simulink model "Main_Simulation_2020a"  (R2020a)
settings: Solver=ode45  StartTime=0.0  StopTime=200  MaxStep=0.01  RelTol=1e-7
values from neighbouring files (symbols this model uses):
  beta = 10    [parameters.m]
  I_g = diag([0.13, 0.16, 0.2])    [parameters.m]
  k1 = 1    [parameters.m]
  k2 = 2    [parameters.m]
  K_p = 10    [parameters.m]
  kp = 16    [parameters.m]
  kv = 6    [parameters.m]
  L = [-(1/2)^(-1/2) -(1/2)^(-1/2) (1/2)^(-1/2)  (1/2)^(-1/2) 0 0 0 0 ... (first row only)    [parameters.m]
  m = 10    [parameters.m]
  M_11 = MRB_11 + MA_11    [parameters.m]
  M_22 = MRB_22 + MA_22    [parameters.m]
  M_q = 10    [parameters.m]
  N_r = 10    [parameters.m]
  r_g = [0 0 0]'    [parameters.m]
  X_u = 10    [parameters.m]
  Y_v = 10    [parameters.m]
  Z_w = 10    [parameters.m]
settings Model: Creator=edward  LastModifiedBy=edward

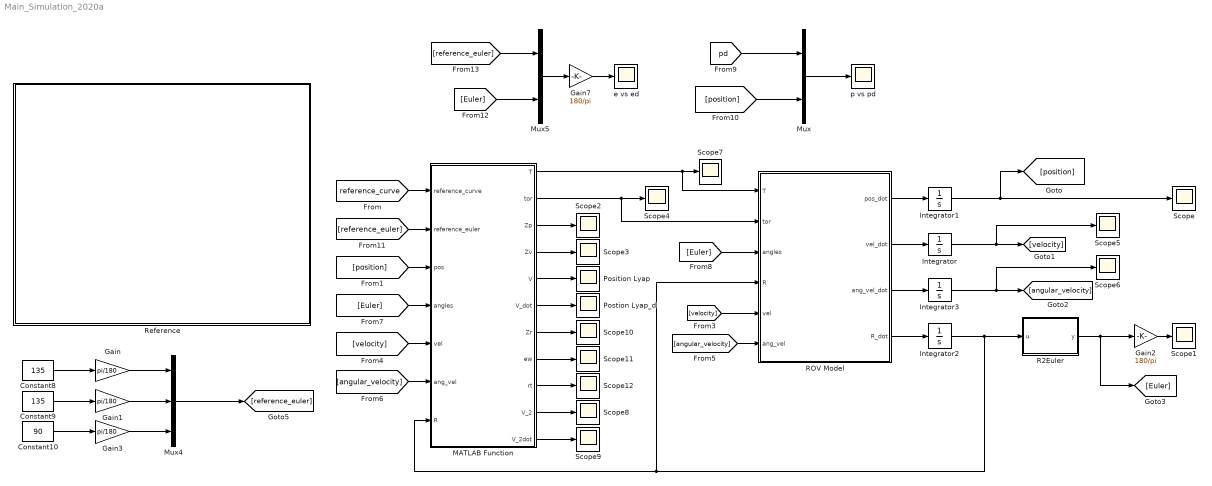
== system Main_Simulation_2020a ==
  Constant10 : Constant  Value=90
  Constant8 : Constant  Value=135
  Constant9 : Constant  Value=135
  Gain : Gain  Gain=pi/180
  Gain1 : Gain  Gain=pi/180
  Gain2 : Gain  Gain=180/pi
  Gain3 : Gain  Gain=pi/180
  Gain7 : Gain  Gain=180/pi
  Integrator : Integrator  InitialCondition=zeros(3,1)
  Integrator1 : Integrator  InitialCondition=[100; 50; -25]
  Integrator2 : Integrator  InitialCondition=eye(3)
  Integrator3 : Integrator  InitialCondition=zeros(3,1)
  MATLAB Function : MATLAB Function  TreatAsAtomicUnit=on
  Mux : Mux  Inputs=2
  Mux4 : Mux  Inputs=3
  Mux5 : Mux  Inputs=2
  Position Lyap : Scope
  Postion Lyap_d : Scope
  R2Euler : MATLAB Function  TreatAsAtomicUnit=on
  ROV Model : MATLAB Function  TreatAsAtomicUnit=on
  Reference : Subsystem
  Scope{,1..12} (13 alike) : Scope
  e vs ed : Scope
  p vs pd : Scope
  wires:
  ROV Model/2(vel_dot) -> Integrator/1
  ROV Model/1(pos_dot) -> Integrator1/1
  Integrator1/1 -> [position], Scope/1
  ROV Model/4(R_dot) -> Integrator2/1
  Integrator2/1 -> R2Euler/1(u), ROV Model/4(R), MATLAB Function/7(R)
  R2Euler/1(y) -> Gain2/1, [Euler]
  Gain2/1 -> Scope1/1
  MATLAB Function/1(T) -> Scope7/1, ROV Model/1(T)
  Integrator/1 -> Scope5/1, [velocity]
  MATLAB Function/3(Zp) -> Scope2/1
  [reference_curve] -> MATLAB Function/1(reference_curve)
  ROV Model/3(ang_vel_dot) -> Integrator3/1
  [position] -> MATLAB Function/3(pos)
  [velocity] -> ROV Model/5(vel)
  [velocity] -> MATLAB Function/5(vel)
  [angular_velocity] -> ROV Model/6(ang_vel)
  [angular_velocity] -> MATLAB Function/6(ang_vel)
  [Euler] -> ROV Model/3(angles)
  [Euler] -> MATLAB Function/4(angles)
  [pd] -> Mux/1
  [position] -> Mux/2
  Mux/1 -> p vs pd/1
  MATLAB Function/5(V) -> Position Lyap/1
  MATLAB Function/4(Zv) -> Scope3/1
  Integrator3/1 -> Scope6/1, [angular_velocity]
  MATLAB Function/6(V_dot) -> Postion Lyap_d/1
  MATLAB Function/2(tor) -> Scope4/1, ROV Model/2(tor)
  Constant8/1 -> Gain/1
  Constant9/1 -> Gain1/1
  Constant10/1 -> Gain3/1
  Gain/1 -> Mux4/1
  Gain1/1 -> Mux4/2
  Gain3/1 -> Mux4/3
  Mux4/1 -> [reference_euler]
  [reference_euler] -> MATLAB Function/2(reference_euler)
  Mux5/1 -> Gain7/1
  [Euler] -> Mux5/2
  [reference_euler] -> Mux5/1
  MATLAB Function/10(V_2) -> Scope8/1
  MATLAB Function/11(V_2dot) -> Scope9/1
  MATLAB Function/7(Zr) -> Scope10/1
  Gain7/1 -> e vs ed/1
  MATLAB Function/8(ew) -> Scope11/1
  MATLAB Function/9(rt) -> Scope12/1

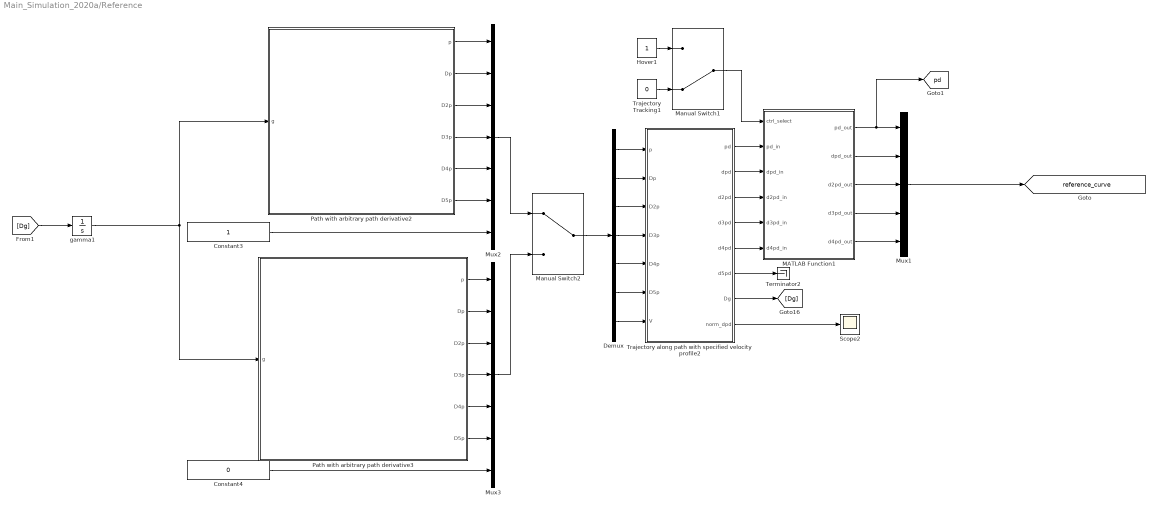
== system Main_Simulation_2020a/Reference ==
  Constant3 : Constant
  Constant4 : Constant  Value=0
  Demux : Demux  Outputs=7
  Hover1 : Constant
  MATLAB Function1 : MATLAB Function  TreatAsAtomicUnit=on
  Manual Switch1 : ManualSwitch  CurrentSetting=0
  Manual Switch2 : ManualSwitch
  Mux1 : Mux  Inputs=5
  Mux2 : Mux  Inputs=7
  Mux3 : Mux  Inputs=7
  Path with arbitrary path derivative2 : MATLAB Function  TreatAsAtomicUnit=on  mask{ra=10, rb=10, a=3, b=3, delta=pi/2, h=0, f=0}
      mask prompts: ra "A"; rb "B"; h "Mean height"; f "Height frequency"
      mask help:
      | x=A*sin(a*g+delta)
      | y=B*sin(b*g)
  Path with arbitrary path derivative3 : MATLAB Function  TreatAsAtomicUnit=on  mask{va=0, h=0}
      mask prompts: va "Radius"; h "Height"
      mask help:
      | x = va*(1 + cos(g))
      | y = va*sin(g)
      | z = 2*va*sin(g/2)
  Scope2 : Scope
  Terminator2 : Terminator
  Trajectory Tracking1 : Constant  Value=0
  Trajectory along path with specified velocity profile2 : MATLAB Function  TreatAsAtomicUnit=on
  gamma1 : Integrator
  tag scope: pd=global, reference_curve=global
  wires:
  Trajectory along path with specified velocity profile2/5(d4pd) -> MATLAB Function1/6(d4pd_in)
  Demux/5 -> Trajectory along path with specified velocity profile2/5(D4p)
  Path with arbitrary path derivative2/5(D4p) -> Mux2/5
  Constant3/1 -> Mux2/7
  MATLAB Function1/2(dpd_out) -> Mux1/2
  MATLAB Function1/3(d2pd_out) -> Mux1/3
  MATLAB Function1/1(pd_out) -> [pd], Mux1/1
  Trajectory along path with specified velocity profile2/2(dpd) -> MATLAB Function1/3(dpd_in)
  Path with arbitrary path derivative2/3(D2p) -> Mux2/3
  Demux/6 -> Trajectory along path with specified velocity profile2/6(D5p)
  MATLAB Function1/4(d3pd_out) -> Mux1/4
  Demux/1 -> Trajectory along path with specified velocity profile2/1(p)
  Trajectory along path with specified velocity profile2/3(d2pd) -> MATLAB Function1/4(d2pd_in)
  Path with arbitrary path derivative3/6(D5p) -> Mux3/6
  Trajectory along path with specified velocity profile2/4(d3pd) -> MATLAB Function1/5(d3pd_in)
  Trajectory along path with specified velocity profile2/1(pd) -> MATLAB Function1/2(pd_in)
  gamma1/1 -> Path with arbitrary path derivative2/1(g), Path with arbitrary path derivative3/1(g)
  MATLAB Function1/5(d4pd_out) -> Mux1/5
  Path with arbitrary path derivative2/6(D5p) -> Mux2/6
  Constant4/1 -> Mux3/7
  Path with arbitrary path derivative3/4(D3p) -> Mux3/4
  Trajectory Tracking1/1 -> Manual Switch1/2
  Manual Switch2/1 -> Demux/1
  Demux/2 -> Trajectory along path with specified velocity profile2/2(Dp)
  Demux/4 -> Trajectory along path with specified velocity profile2/4(D3p)
  Mux3/1 -> Manual Switch2/2
  Mux2/1 -> Manual Switch2/1
  Trajectory along path with specified velocity profile2/8(norm_dpd) -> Scope2/1
  Path with arbitrary path derivative3/3(D2p) -> Mux3/3
  Trajectory along path with specified velocity profile2/7(Dg) -> [Dg]
  Hover1/1 -> Manual Switch1/1
  Demux/3 -> Trajectory along path with specified velocity profile2/3(D2p)
  Path with arbitrary path derivative2/2(Dp) -> Mux2/2
  Trajectory along path with specified velocity profile2/6(d5pd) -> Terminator2/1
  Path with arbitrary path derivative3/2(Dp) -> Mux3/2
  Path with arbitrary path derivative3/1(p) -> Mux3/1
  Path with arbitrary path derivative2/1(p) -> Mux2/1
  Manual Switch1/1 -> MATLAB Function1/1(ctrl_select)
  [Dg] -> gamma1/1
  Demux/7 -> Trajectory along path with specified velocity profile2/7(V)
  Path with arbitrary path derivative2/4(D3p) -> Mux2/4
  Path with arbitrary path derivative3/5(D4p) -> Mux3/5
  Mux1/1 -> [reference_curve]

== matlab function Main_Simulation_2020a/Reference/MATLAB Function1 ==
  data: ctrl_select input; pd_out output; pd_in input; dpd_in input; d2pd_in input; d3pd_in input; d4pd_in input; dpd_out output; d2pd_out output; d3pd_out output; d4pd_out output
function [pd_out, dpd_out, d2pd_out, d3pd_out, d4pd_out] = hover_ref(ctrl_select,pd_in, dpd_in, d2pd_in, d3pd_in, d4pd_in)

pd_out      = (1 - ctrl_select)*pd_in;
dpd_out     = (1 - ctrl_select)*dpd_in;
d2pd_out    = (1 - ctrl_select)*d2pd_in;
d3pd_out    = (1 - ctrl_select)*d3pd_in;
d4pd_out    = (1 - ctrl_select)*d4pd_in;
    
if ctrl_select == 1
    pd_out(3) = -1.7;
end

== matlab function Main_Simulation_2020a/Reference/Path with arbitrary path derivative2 ==
  data: g input; ra parameter; rb parameter; a parameter; b parameter; delta parameter; p output; Dp output; D2p output; D3p output; D4p output; D5p output; h parameter size=1; f parameter
function [p,Dp,D2p,D3p,D4p,D5p] = path(g,ra,rb,a,b,delta,h,f)
%#codegen

% syms a b g delta ra rb
% p = [ra*sin(a*g+delta)/(sin(b*g)^2+1);
%      rb*sin(b*g)/(sin(b*g)^2+1)]
% diff(p,g)
% diff(p,g,2)
% diff(p,g,3)

p = [ra*sin(a*g+delta);
     rb*sin(b*g);
     h + 0.5*sin(f*g)];
 
Dp = [a*ra*cos(delta + a*g);
      b*rb*cos(b*g);
      0.5*f*cos(f*g)];
      
D2p = [-a^2*ra*sin(delta + a*g);
       -b^2*rb*sin(b*g);
       -0.5*f^2*sin(f*g)];
 
D3p = [-a^3*ra*cos(delta + a*g);
       -b^3*rb*cos(b*g);
       -0.5*f^3*cos(f*g)];
     
D4p = [a^4*ra*sin(delta + a*g);
       b^4*rb*sin(b*g);
       0.5*f^4*sin(f*g)];
 
D5p = [a^5*ra*cos(delta + a*g);
       b^5*rb*cos(b*g);
       0.5*f^5*cos(f*g)];

== matlab function Main_Simulation_2020a/Reference/Path with arbitrary path derivative3 ==
  data: g input; p output; Dp output; D2p output; D3p output; D4p output; D5p output; va parameter size=1; h parameter
function [p,Dp,D2p,D3p,D4p,D5p] = path(g,va, h)
%#codegen

% syms g va
% p = [va*sin(g);
%      2*va*sin(g/2);
%      va*(1 + cos(g))];
% diff(p,g)
% diff(p,g,2)
% diff(p,g,3)

p = [va*sin(g);
     2*va*sin(g/2);
     va*(1 + cos(g)) - h];

Dp = [va*cos(g);
       va*cos(g/2);
       -va*sin(g)];
         
D2p = [-va*sin(g);
       -(va/2)*sin(g/2);
       -va*cos(g)];

D3p = [-va*cos(g);
       -(va/4)*cos(g/2);
       va*sin(g)];
        
D4p = [va*sin(g);
       (va/8)*sin(g/2);
       va*cos(g)];
    
D5p = [va*cos(g);
        (va/16)*cos(g/2);
        -va*sin(g)];

== matlab function Main_Simulation_2020a/Reference/Trajectory along path with specified velocity profile2 ==
  data: pd output size=3; dpd output size=3; d2pd output size=3; d3pd output; d4pd output; d5pd output; Dg output; p input size=3; Dp input size=3; D2p input size=3; D3p input size=3; D4p input size=3; D5p input size=3; V input; norm_dpd output
function [pd,dpd,d2pd,d3pd,d4pd,d5pd,Dg,norm_dpd] = trajectory(p,Dp,D2p,D3p,D4p,D5p,V)
%#codegen

norm_Dp = norm(Dp);

% Parameter velocity is V times the inverse of the 
% norm of path derivative with respect to the parameter
Dg = V/norm_Dp;

% Checked
D2g = -V*(Dp'*D2p)/norm_Dp^3*Dg;

% Checked
D3g = -V/norm_Dp^3*((Dp'*D2p)*D2g + Dg^2*(norm(D2p)^2 + Dp'*D3p - 3*(Dp'*D2p)^2/norm_Dp^2));

% Checked
Aux = 2*(     (Dp'*D2p)*Dg*norm(D2p)^2/norm_Dp^2 ...
            + (Dp'*D2p)*(Dp'*D3p)*Dg/norm_Dp^2 ...
            - (Dp'*D2p)^3*Dg/norm_Dp^4);

% As seen before, Aux variable is divided into 3 different components
% In the next step, we compute the derivative of each component 

% Checked
J1 = ((norm(D2p)^2*Dg^2 + (Dp'*D3p)*Dg^2 + (Dp'*D2p)*D2g))*norm(D2p)^2/norm_Dp^2 ...
        + (Dp'*D2p)*Dg*(2*(D3p'*D2p)*Dg*norm_Dp^2 - 2*norm(D2p)^2*(D2p'*Dp)*Dg)/norm_Dp^4;

% Checked
J2_aux = norm(D2p)^2*(Dp'*D3p)*Dg^2 + (Dp'*D3p)^2*Dg^2 + (Dp'*D2p)*(D2p'*D3p)*Dg^2 + (Dp'*D2p)*(Dp'*D4p)*Dg^2 + (Dp'*D2p)*(Dp'*D3p)*D2g;

% Checked
J2 = -2*(D2p'*Dp)*Dg/norm_Dp^4*(Dp'*D2p)*(Dp'*D3p)*Dg + 1/norm_Dp^2*(J2_aux);

% Checked
J3 = -1/norm_Dp^4*(3*(Dp'*D2p)^2*(norm(D2p)^2 + (Dp'*D3p))*Dg^2 + (Dp'*D2p)^3*D2g - 4*(Dp'*D2p)^4*Dg^2/norm_Dp^2);

% Checked
Aux_der = 2*(J1 + J2 + J3);

% Checked
D4g_aux1 = (Dp'*D2p)*D2g + Dg^2*(norm(D2p)^2 + Dp'*D3p - 3*(Dp'*D2p)^2/norm_Dp^2);

% Checked
D4g_aux2 = (norm(D2p)^2 + Dp'*D3p)*D2g*Dg ... % T1
            + (Dp'*D2p)*D3g ... % T2
            +2*Dg*D2g*(norm(D2p)^2 + Dp'*D3p - 3*(Dp'*D2p)^2/norm_Dp^2) ... % T3
            +Dg^2*(2*(D3p'*D2p)*Dg + (D2p'*D3p)*Dg + (Dp'*D4p)*Dg - 3*Aux);

% Checked
D4g = 3*V*(Dp'*D2p)*Dg/norm_Dp^5*D4g_aux1 - V/norm_Dp^3*D4g_aux2;

% Checked
D4g_aux1_der = (norm(D2p)^2 + Dp'*D3p)*D2g*Dg + (Dp'*D2p)*D3g ...
                + 2*Dg*D2g*(norm(D2p)^2 + Dp'*D3p - 3*(Dp'*D2p)^2/norm_Dp^2) ...
                + Dg^2*(2*(D3p'*D2p)*Dg + (D2p'*D3p)*Dg + (Dp'*D4p)*Dg - 3*Aux);

% Checked
T1_der = (2*(D3p'*D2p)*Dg + (D2p'*D3p)*Dg + (Dp'*D4p)*Dg)*D2g*Dg + (norm(D2p)^2 + Dp'*D3p)*(D3g*Dg + D2g^2);

% Checked
T2_der = norm(D2p)^2*D3g*Dg + (Dp'*D3p)*D3g*Dg + (Dp'*D2p)*D4g;

% Checked
T3_der = 2*(D2g^2 + Dg*D3g)*(norm(D2p)^2 + Dp'*D3p - 3*(Dp'*D2p)^2/norm_Dp^2)...
        + 2*Dg*D2g*(2*(D3p'*D2p)*Dg + (D2p'*D3p)*Dg + (Dp'*D4p)*Dg - 3*Aux);

% Checked
T4_der = 2*Dg*D2g*(2*(D3p'*D2p)*Dg + (D2p'*D3p)*Dg + (Dp'*D4p)*Dg - 3*Aux) ...
            + Dg^2*(3*(D4p'*D2p)*Dg^2 + 3*norm(D3p)^2*Dg^2 + 3*D3p'*D2p*D2g + (D2p'*D4p)*Dg^2 + Dp'*D5p*Dg^2 + Dp'*D4p*D2g - 3*Aux_der);

% Checked
D4g_aux2_der = T1_der + T2_der + T3_der + T4_der;
  
D5g =   3*V*((norm(D2p)^2*Dg^2 + Dp'*D3p*Dg^2 + Dp'*D2p*D2g)/norm_Dp^5 ...
        - 5*((Dp'*D2p)^2*Dg^2)/norm_Dp^7)*D4g_aux1 ...
        + 3*V*(Dp'*D2p)*Dg/norm_Dp^5*D4g_aux1_der + 3*V*(Dp'*D2p)*Dg/norm_Dp^5*D4g_aux2 ...
        -V/norm_Dp^3*D4g_aux2_der;
    
pd      = p;
dpd     = Dp*Dg;
d2pd    = D2p*Dg^2 + Dp*D2g;
d3pd    = D3p*Dg^3 + 3*D2p*D2g*Dg + Dp*D3g;
d4pd    = D4p*Dg^4 + 6*D3p*Dg^2*D2g + D2p*(4*D3g*Dg + 3*D2g^2) + Dp*D4g;
d5pd    = D5p*Dg^5 + 10*D4p*Dg^3*D2g + 15*D3p*D2g^2*Dg + 10*D3p*Dg^2*D3g + 5*D2p*D4g*Dg + 10*D2p*D3g*D2g + Dp*D5g;

norm_dpd = norm(dpd);

== matlab function Main_Simulation_2020a/ROV Model ==
  data: T input size=3; tor input size=3; pos_dot output size=3; angles input size=3; R input; vel_dot output size=3; ang_vel_dot output size=3; vel input size=3; R_dot output size=[3 3]; ang_vel input size=3; L parameter size=[6 8]; M_11 parameter size=[3 3]; M_22 parameter size=[3 3]; I_g parameter size=[3 3]; r_g parameter size=3; X_u parameter size=1; Y_v parameter size=1; Z_w parameter size=1; K_p parameter size=1; M_q parameter size=1; N_r parameter size=1; m parameter size=1
function [pos_dot,vel_dot,ang_vel_dot,R_dot] = fcn(T,tor,angles,R,vel,ang_vel,L,M_11,M_22,I_g,r_g,X_u,Y_v,Z_w, K_p, M_q, N_r, m)

roll = angles(1);
pitch = angles(2);
yaw = angles(3);

v_surge = vel(1);
v_sway = vel(2);
v_heave = vel(3);

w_roll = ang_vel(1);
w_pitch = ang_vel(2);
w_yaw = ang_vel(3);


CRB_11 = zeros(3,3);
CRB_12 = -m*Skew(vel)-m*Skew(Skew(ang_vel)*r_g);
CRB_21 = -m*Skew(vel)-m*Skew(Skew(ang_vel)*r_g);
CRB_22 = m*Skew(Skew(vel)*r_g)-Skew(I_g*ang_vel);
   
aux_a = diag([X_u, Y_v, Z_w])*vel;
aux_b = diag([K_p, M_q, N_r])*ang_vel;

CA_11 = zeros(3,3);
CA_12 = Skew(aux_a);
CA_21 = Skew(aux_a);
CA_22 = Skew(aux_b);

C_11 = CRB_11 + CA_11;
C_12 = CRB_12 + CA_12;
C_21 = CRB_21 + CA_21;
C_22 = CRB_22 + CA_22;

Xu = 10;
Yv = 10;
Zw = 10;
Kp = 10;
Mq = 10;
Nr = 10;
Xuu = 10;
Yvv = 10;
Zww = 10;
Kpp = 10;
Mqq = 10;
Nrr = 10; 

Dl_11 = diag([Xu, Yv, Zw]);
Dl_22 = diag([Kp, Mq, Nr]);

Dq_11 = diag([Xuu*abs(v_surge), Yvv*abs(v_sway), Zww*abs(v_heave)]);
Dq_22 = diag([Kpp*abs(w_roll), Mqq*abs(w_pitch), Nrr*abs(w_yaw)]);

D_11 = Dl_11 + Dq_11;
D_22 = Dl_22 + Dq_22;


W = 9.81*m;
B = 1000*9.81*0.0480;
g_v = (W-B)*[sin(pitch);
     -cos(pitch)*sin(roll);
     -cos(pitch)*cos(roll)];

pos_dot = R*vel;

R_dot = R*Skew(ang_vel);

vel_dot = M_11\(T - [C_11 C_12]*[vel; ang_vel] - D_11*vel - g_v);

ang_vel_dot = M_22\(tor - [C_21 C_22]*[vel; ang_vel] - D_22*ang_vel);

== matlab function Main_Simulation_2020a/R2Euler ==
  data: u input; y output
function y = fcn(u)
y = rotm2eul(u, 'XYZ')';

== matlab function Main_Simulation_2020a/MATLAB Function ==
  data: reference_curve input size=15; reference_euler input size=3; pos input size=3; angles input size=3; vel input size=3; ang_vel input size=3; R input size=[3 3]; T output size=3; tor output size=3; Zp output size=3; Zv output; V output size=1; M_11 parameter size=[3 3]; m parameter size=1; M_q parameter size=1; N_r parameter size=1; r_g parameter size=3; X_u parameter size=1; Y_v parameter size=1; Z_w parameter size=1; I_g parameter size=[3 3]; K_p parameter size=1; k1 parameter size=1; k2 parameter size=1; kp parameter size=1; kv parameter size=1; beta parameter size=1; V_dot output size=1; Zr output size=[3 3]; ew output; rt output; V_2 output size=1; M_22 parameter size=[3 3]; V_2dot output size=1
function [T,tor,Zp,Zv,V,V_dot,Zr,ew,rt,V_2,V_2dot] = fcn(reference_curve,reference_euler,pos,angles,vel,ang_vel,R,M_11,m, M_q, N_r, r_g, X_u, Y_v, Z_w, I_g, K_p, k1, k2, kp, kv, beta, M_22)

pd      = reference_curve(1:3);
dpd     = reference_curve(4:6);
d2pd    = reference_curve(7:9);

roll = angles(1);
pitch = angles(2);

Zp = pos - pd;
Zv = R*vel - dpd;

v_surge = vel(1);
v_sway = vel(2);
v_heave = vel(3);

w_roll = ang_vel(1);
w_pitch = ang_vel(2);
w_yaw = ang_vel(3);

CRB_11 = zeros(3,3);
CRB_12 = -m*Skew(vel)-m*Skew(Skew(ang_vel)*r_g);
CRB_21 = -m*Skew(vel)-m*Skew(Skew(ang_vel)*r_g);
CRB_22 = m*Skew(Skew(vel)*r_g)-Skew(I_g*ang_vel);
   
aux_a = diag([X_u, Y_v, Z_w])*vel;
aux_b = diag([K_p, M_q, N_r])*ang_vel;

CA_11 = zeros(3,3);
CA_12 = Skew(aux_a);
CA_21 = Skew(aux_a);
CA_22 = Skew(aux_b);
    
C_11 = CRB_11 + CA_11;
C_12 = CRB_12 + CA_12;
C_21 = CRB_21 + CA_21;
C_22 = CRB_22 + CA_22;

Xu = 10;
Yv = 10;
Zw = 10;
Kp = 10;
Mq = 10;
Nr = 10;
Xuu = 10;
Yvv = 10;
Zww = 10;
Kpp = 10;
Mqq = 10;
Nrr = 10; 

Dl_11 = diag([Xu, Yv, Zw]);
Dl_22 = diag([Kp, Mq, Nr]);

Dq_11 = diag([Xuu*abs(v_surge), Yvv*abs(v_sway), Zww*abs(v_heave)]);
Dq_22 = diag([Kpp*abs(w_roll), Mqq*abs(w_pitch), Nrr*abs(w_yaw)]);

D_11 = Dl_11 + Dq_11;
D_22 = Dl_22 + Dq_22;


W = 9.81*m;
B = 1000*9.81*0.0480;
g_v = (W-B)*[       sin(pitch);
                -cos(pitch)*sin(roll);
                -cos(pitch)*cos(roll)];
 
%vel_dot = M_11\(T - [C_11 C_12]*[vel; ang_vel] - D_11*vel - g_v);

T = ([C_11 C_12]*[vel; ang_vel] + D_11*vel + g_v + M_11*R'*(d2pd - R*Skew(ang_vel)*vel - k1*Zp - k2*Zv));

V = kp/2*(Zp'*Zp) + kv/2*(Zv'*Zv) + beta/2*(Zp'*Zv);

V_dot = -k1*beta/2*(Zp')*Zp - (k2*kv - beta/2)*(Zv')*Zv;

Rd = eul2rotm(reference_euler','XYZ');

Zr = R*Rd';
Zr_dot = R*Skew(ang_vel)*Rd';

quat = rotm2quat(Zr);

st = quat(1);
rt = (quat(2:4))';
st_dot = -0.5*rt'*Rd*ang_vel;
rt_dot = 0.5*(st*eye(3) + Skew(rt))*Rd*ang_vel;

wd = -st*Rd'*rt;
wd_dot = -st_dot*Rd'*rt - st*Rd'*rt_dot;
ew = ang_vel - wd;

tor = M_22*(wd_dot - ew - st*Rd*rt) + [C_21 C_22]*[vel; ang_vel] + D_22*ang_vel;

V_1 = (rt')*rt;

V_1dot = -st^2*((Rd*rt)')*Rd*rt + st*rt'*Rd'*ew;

V_2 = (rt')*rt + 0.5*(ew')*ew;

V_2dot = -st^2*((Rd*rt)')*Rd*rt - (ew')*ew;
